simulink model "k1visitmyt"  (Simulink 8.6)
settings: Solver=ode45  StartTime=0.0  StopTime=10.0  RelTol=1e-3
libraries: cdsIPCx x21, cdsTP x5, cdsCDI64 x4, cdsCDO64 x4, BIO_CD_ENCODE_MASTER x4, BIO_CD_DECODE_MASTER x4, CHK_DIO x4, VIS_LIB x3, dac x2, cdsAdcx0 x1, cdsAdcx1 x1, cdsAdcx2 x1
settings Model: Creator=controls  LastModifiedBy=controls
settings DataIOCC: SignalLoggingSaveFormat=Dataset
settings OptimizationCC: ExpressionDepthLimit=128
settings DebuggingCC: UnderspecifiedInitializationDetection=Simplified  MergeDetectMultiDrivingBlocksExec=error  SolverPrmCheckMsg=none  FcnCallInpInsideContextMsg=EnableAllAsError  StateNameClashWarn=none
settings GRTTargetCC: CombineOutputUpdateFcns=on  GRTInterface=off

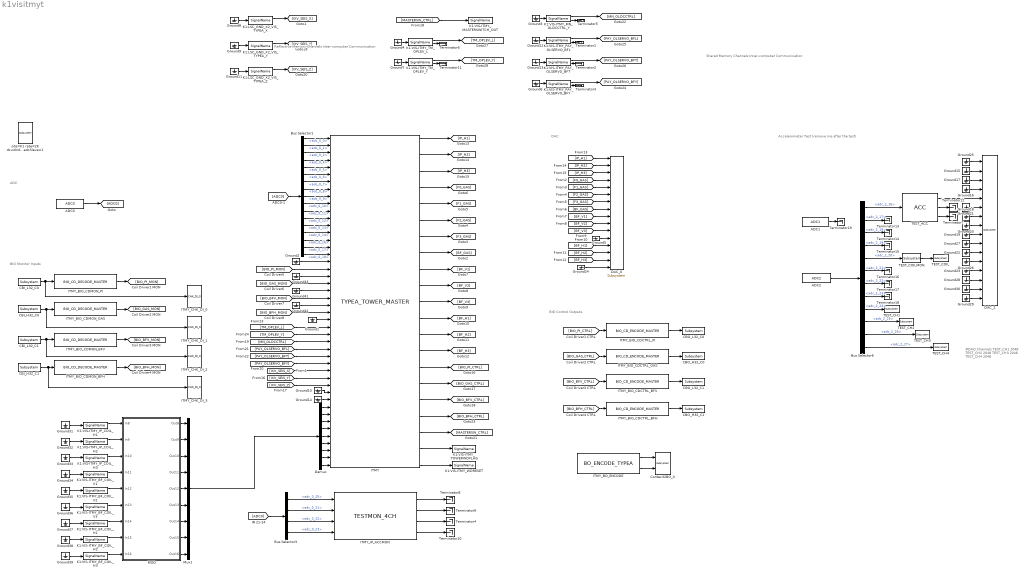
== system k1visitmyt ==
  note: BIO Monitor Inputs
  note: BIO Control Outputs
  note: DAC
  note: ADC
  note: Reflective Memory Channels
      | Inter-computer Communication
  note: Shared Memory Channels
      | Inner-computer Communication
  note: Accelerometer Test (remove me after the test)
  note: #DAQ Channels
      |
      | TEST_CH1 2048
      | TEST_CH2 2048
      | TEST_CH3 2048
      | TEST_CH4 2048
  ADC0 : cdsAdcx0/ADC0  Tag=cdsAdc  Description=|
      | type-GSC_16AI64SSA
      | card_num=0
      settings: AttributesFormatString=%<Description>\n%<Tag>
  ADC1 : cdsAdcx1/ADC1  Tag=cdsAdc  Description=|
      | type-GSC_16AI64SSA
      | card_num=1
      settings: AttributesFormatString=%<Description>\n%<Tag>
  ADC2 : cdsAdcx2/ADC2  Tag=cdsAdc  Description=|
      | type-GSC_16AI64SSA
      | card_num=2
      settings: AttributesFormatString=%<Description>\n%<Tag>
  Bus Selector1 : BusSelector  OutputSignals=adc_0_0,adc_0_1,adc_0_2,adc_0_4,adc_0_5,adc_0_6,adc_0_7,adc_0_8,adc_0_9,adc_0_10,adc_0_11,adc_0_12,adc_0_13,adc_0_14,adc_0_16,adc_0_17,adc_0_18
  Bus Selector3 : BusSelector  OutputSignals=adc_0_20,adc_0_21,adc_0_22,adc_0_23
  Bus Selector6 : BusSelector  Description=ADC Selector  OutputSignals=adc_2_16,adc_2_17,adc_2_18,adc_2_19,adc_2_20,adc_2_21,adc_2_22,adc_2_23,adc_2_24,adc_2_25,adc_2_26,adc_2_27
      settings: AttributesFormatString=%<Description>
  CBI_H32_C0 : cdsCDI64/Subsystem  Tag=cdsCDI64  Description=card_num=1
      settings: AttributesFormatString=%<Tag>\n%<Description>
  CBI_H32_C1 : cdsCDI64/Subsystem  Tag=cdsCDI64  Description=card_num=3
      settings: AttributesFormatString=%<Tag>\n%<Description>
  CBI_L32_C0 : cdsCDI64/Subsystem  Tag=cdsCDI64  Description=card_num=0
      settings: AttributesFormatString=%<Tag>\n%<Description>
  CBI_L32_C1 : cdsCDI64/Subsystem  Tag=cdsCDI64  Description=card_num=2
      settings: AttributesFormatString=%<Tag>\n%<Description>
  CBO_H32_C0 : cdsCDO64/Subsystem  Tag=cdsCDO64  Description=card_num=1
      settings: AttributesFormatString=%<Tag>\n%<Description>
  CBO_H32_C1 : cdsCDO64/Subsystem  Tag=cdsCDO64  Description=card_num=3
      settings: AttributesFormatString=%<Tag>\n%<Description>
  CBO_L32_C0 : cdsCDO64/Subsystem  Tag=cdsCDO64  Description=card_num=0
      settings: AttributesFormatString=%<Tag>\n%<Description>
  CBO_L32_C1 : cdsCDO64/Subsystem  Tag=cdsCDO64  Description=card_num=2
      settings: AttributesFormatString=%<Tag>\n%<Description>
  Contec32BO_0 : cdsCDO32/Subsystem  Tag=cdsCDO32  Description=Contec32 bit binary output module driver
      settings: AttributesFormatString=%<Tag>
  DAC_0 : dac/Subsystem  Description=|
      | type=GSC_16AO16,
      | card_num=0
      settings: AttributesFormatString=%<Description>
  DAC_2 : dac/Subsystem  Description=|
      | type=GSC_16AO16,
      | card_num=2
      settings: AttributesFormatString=%<Description>
  Demux : Demux  Outputs=9
  Ground{1..39,41..43} (42 alike) : Ground
  ITMY : TYPEA_MASTER/TYPEA_TOWER_MASTER
  ITMY_BIO_CDCTRL_BFH : BIO_CD_ENCODE_MASTER/BIO_CD_ENCODE_MASTER
  ITMY_BIO_CDCTRL_BFV : BIO_CD_ENCODE_MASTER/BIO_CD_ENCODE_MASTER
  ITMY_BIO_CDCTRL_GAS : BIO_CD_ENCODE_MASTER/BIO_CD_ENCODE_MASTER
  ITMY_BIO_CDCTRL_PI : BIO_CD_ENCODE_MASTER/BIO_CD_ENCODE_MASTER
  ITMY_BIO_CDMON_BFH : BIO_CD_DECODE_MASTER/BIO_CD_DECODE_MASTER
  ITMY_BIO_CDMON_BFV : BIO_CD_DECODE_MASTER/BIO_CD_DECODE_MASTER
  ITMY_BIO_CDMON_GAS : BIO_CD_DECODE_MASTER/BIO_CD_DECODE_MASTER
  ITMY_BIO_CDMON_PI : BIO_CD_DECODE_MASTER/BIO_CD_DECODE_MASTER
  ITMY_BO_ENCODE : BO_TYPEA_MASTER/BO_ENCODE_TYPEA
  ITMY_CHK_DI_{0..3} (4 alike) : CHK_DIO/CHK_DI_0
  ITMY_IP_ACCMON : TESTMON_4CH_MASTER/TESTMON_4CH
  K1:LSC_GND_X2_VIS_TYPEA_X : cdsIPCx/SignalName  Tag=cdsIPCx_RFM  Description=card=1
      settings: AttributesFormatString=%<Description>\n%<Tag>
  K1:LSC_GND_X2_VIS_TYPEA_Y : cdsIPCx/SignalName  Tag=cdsIPCx_RFM  Description=card=1
      settings: AttributesFormatString=%<Description>\n%<Tag>
  K1:LSC_GND_X2_VIS_TYPEA_Z : cdsIPCx/SignalName  Tag=cdsIPCx_RFM  Description=card=1
      settings: AttributesFormatString=%<Description>\n%<Tag>
  K1:VIS-ITMY_BF_COIL_H1 : cdsIPCx/SignalName  Tag=cdsIPCx_SHMEM  Description=Inter-Process Communication via Shared memory.
      settings: AttributesFormatString=%<Tag>
  K1:VIS-ITMY_BF_COIL_H2 : cdsIPCx/SignalName  Tag=cdsIPCx_SHMEM  Description=Inter-Process Communication via Shared memory.
      settings: AttributesFormatString=%<Tag>
  K1:VIS-ITMY_BF_COIL_H3 : cdsIPCx/SignalName  Tag=cdsIPCx_SHMEM  Description=Inter-Process Communication via Shared memory.
      settings: AttributesFormatString=%<Tag>
  K1:VIS-ITMY_BF_COIL_V1 : cdsIPCx/SignalName  Tag=cdsIPCx_SHMEM  Description=Inter-Process Communication via Shared memory.
      settings: AttributesFormatString=%<Tag>
  K1:VIS-ITMY_BF_COIL_V2 : cdsIPCx/SignalName  Tag=cdsIPCx_SHMEM  Description=Inter-Process Communication via Shared memory.
      settings: AttributesFormatString=%<Tag>
  K1:VIS-ITMY_BF_COIL_V3 : cdsIPCx/SignalName  Tag=cdsIPCx_SHMEM  Description=Inter-Process Communication via Shared memory.
      settings: AttributesFormatString=%<Tag>
  K1:VIS-ITMY_IP_COIL_H1 : cdsIPCx/SignalName  Tag=cdsIPCx_SHMEM  Description=Inter-Process Communication via Shared memory.
      settings: AttributesFormatString=%<Tag>
  K1:VIS-ITMY_IP_COIL_H2 : cdsIPCx/SignalName  Tag=cdsIPCx_SHMEM  Description=Inter-Process Communication via Shared memory.
      settings: AttributesFormatString=%<Tag>
  K1:VIS-ITMY_IP_COIL_H3 : cdsIPCx/SignalName  Tag=cdsIPCx_SHMEM  Description=Inter-Process Communication via Shared memory.
      settings: AttributesFormatString=%<Tag>
  K1:VIS-ITMY_MASTERSWITCH_OUT : cdsIPCx/SignalName  Tag=cdsIPCx_SHMEM  Description=Inter-Process Communication via Shared memory.
      settings: AttributesFormatString=%<Tag>
  K1:VIS-ITMY_MN_OLDCCTRL_Y : cdsIPCx/SignalName  Tag=cdsIPCx_SHMEM  Description=Inter-Process Communication via Shared memory.
      settings: AttributesFormatString=%<Tag>
  K1:VIS-ITMY_PAY_OLSERVO_BFL : cdsIPCx/SignalName  Tag=cdsIPCx_SHMEM  Description=Inter-Process Communication via Shared memory.
      settings: AttributesFormatString=%<Tag>
  K1:VIS-ITMY_PAY_OLSERVO_BFT : cdsIPCx/SignalName  Tag=cdsIPCx_SHMEM  Description=Inter-Process Communication via Shared memory.
      settings: AttributesFormatString=%<Tag>
  K1:VIS-ITMY_PAY_OLSERVO_BFY : cdsIPCx/SignalName  Tag=cdsIPCx_SHMEM  Description=Inter-Process Communication via Shared memory.
      settings: AttributesFormatString=%<Tag>
  K1:VIS-ITMY_TM_OPLEV_L : cdsIPCx/SignalName  Tag=cdsIPCx_SHMEM  Description=Inter-Process Communication via Shared memory.
      settings: AttributesFormatString=%<Tag>
  K1:VIS-ITMY_TM_OPLEV_Y : cdsIPCx/SignalName  Tag=cdsIPCx_SHMEM  Description=Inter-Process Communication via Shared memory.
      settings: AttributesFormatString=%<Tag>
  K1:VIS-ITMY_TOWERWDFLAG : cdsIPCx/SignalName  Tag=cdsIPCx_SHMEM  Description=Inter-Process Communication via Shared memory.
      settings: AttributesFormatString=%<Tag>
  K1:VIS-ITMY_WDRESET : cdsIPCx/SignalName  Tag=cdsIPCx_SHMEM  Description=Inter-Process Communication via Shared memory.
      settings: AttributesFormatString=%<Tag>
  MOD : Subsystem  Tag=top_names
  Mux1 : Mux  Inputs=9
  TEST_ACC : VIS_LIB/ACC
  TEST_CH{1..4} (4 alike) : cdsTP/Subsystem  Tag=Test Point
      settings: AttributesFormatString=%<Tag>
  TEST_COIL : cdsTP/Subsystem  Tag=Test Point
      settings: AttributesFormatString=%<Tag>
  TEST_COILMON : cdsEpicsOut/Subsystem  Tag=cdsEpicsOutput  Description=|
      | Purpose:                                          
      | Output a FE signal to an EPICS channel.           
      |                                                   
      | Operation:                                        
      | Takes input value and passes it to EPICS record.  
      |                                                   
      | Usage:                                            
      | Name the part with the desired EPICS rrecord name.
      settings: AttributesFormatString=%<Tag>
  Terminator{1..19} (19 alike) : Terminator
  site=K1 rate=2K dcuid=62 host=k1iy1 specific_cpu=3 adcSlave=1 : cdsParameters/Subsystem  Tag=cdsParameters  Description=|
      | Purpose:                                                                                                                                                                                                                                
      | Provide system parameters to the FE code generator to properly configure the generated EPICS names, rep rate of the FE controller, and the Data Acquisition node ID for proper storage of data from this FE controller.                 
      |                                                                                                                                                                                                                                         
      | Useage:                                                                                                                                                                                                                                 
      | The part NAME field is used to identify the FE parameters. It must be of the form:                                                                                                                                                      
      | site=                                                                                                                                                                                                                                   
      | rate=                                                                                                                                                                                                                                   
      | dcuid=                                                                                                                                                                                                                                  
      |                                                                                                                                                                                                                                         
      | Where:                                                                                                                                                                                                                                  
      | site= argument may be H1, H2, L1, M1, G1, either as a single argument or multiple, for example site=H1,H2. These are the only names allowed. These will become the first two characters of all EPICS and signal names (for example G1:).
      |                                                                                                                                                                                                                                         
      | rate= may be 2K, 16K, 32K, or 64K                                                                                                                                                                                                       
      |                                                                                                                                                                                                                                         
      | dcuid= is site specific ie it must be unique at each site.
      settings: AttributesFormatString=%<Tag>
  wires:
  ADC0/1 -> [ADC0]
  ITMY/4 -> [F0_GAS]
  ITMY/5 -> [F1_GAS]
  ITMY/8 -> [BF_GAS]
  ITMY/7 -> [F3_GAS]
  ITMY/6 -> [F2_GAS]
  ITMY/9 -> [BF_V1]
  ITMY/10 -> [BF_V2]
  ITMY/11 -> [BF_V3]
  ITMY/12 -> [BF_H1]
  ITMY/13 -> [BF_H2]
  ITMY/14 -> [BF_H3]
  [BF_H2] -> DAC_0/14
  [BF_V3] -> DAC_0/11
  [BF_H3] -> DAC_0/15
  [BF_V1] -> DAC_0/9
  [BF_H1] -> DAC_0/13
  [BF_V2] -> DAC_0/10
  ITMY/1 -> [IP_H1]
  ITMY/2 -> [IP_H2]
  ITMY/3 -> [IP_H3]
  CBI_H32_C0/1 -> ITMY_CHK_DI_1/1, ITMY_BIO_CDMON_GAS/1
  CBI_L32_C1/1 -> ITMY_CHK_DI_2/1, ITMY_BIO_CDMON_BFV/1
  CBI_L32_C0/1 -> ITMY_CHK_DI_0/1, ITMY_BIO_CDMON_PI/1
  CBI_H32_C1/1 -> ITMY_CHK_DI_3/1, ITMY_BIO_CDMON_BFH/1
  ITMY_BIO_CDCTRL_BFH/1 -> CBO_H32_C1/1
  ITMY_BIO_CDCTRL_PI/1 -> CBO_L32_C0/1
  ITMY_BIO_CDCTRL_GAS/1 -> CBO_H32_C0/1
  ITMY_BIO_CDCTRL_BFV/1 -> CBO_L32_C1/1
  [BIO_PI_CTRL] -> ITMY_BIO_CDCTRL_PI/1
  [BIO_GAS_CTRL] -> ITMY_BIO_CDCTRL_GAS/1
  [BIO_BFV_CTRL] -> ITMY_BIO_CDCTRL_BFV/1
  ITMY_BIO_CDMON_PI/1 -> [BIO_PI_MON]
  ITMY_BIO_CDMON_GAS/1 -> [BIO_GAS_MON]
  ITMY_BIO_CDMON_BFH/1 -> [BIO_BFH_MON]
  ITMY_BIO_CDMON_BFV/1 -> [BIO_BFV_MON]
  [BIO_BFH_CTRL] -> ITMY_BIO_CDCTRL_BFH/1
  [IP_H1] -> DAC_0/1
  [IP_H2] -> DAC_0/2
  [IP_H3] -> DAC_0/3
  [F0_GAS] -> DAC_0/4
  [F1_GAS] -> DAC_0/5
  [F2_GAS] -> DAC_0/6
  [F3_GAS] -> DAC_0/7
  [BF_GAS] -> DAC_0/8
  [ADC0] -> Bus Selector3/1
  Bus Selector3/2 -> ITMY_IP_ACCMON/2  "<adc_0_21>"
  Bus Selector3/1 -> ITMY_IP_ACCMON/1  "<adc_0_20>"
  Bus Selector3/3 -> ITMY_IP_ACCMON/3  "<adc_0_22>"
  Bus Selector3/4 -> ITMY_IP_ACCMON/4  "<adc_0_23>"
  ITMY_IP_ACCMON/3 -> Terminator4/1
  ITMY_IP_ACCMON/4 -> Terminator10/1
  ITMY_IP_ACCMON/1 -> Terminator8/1
  ITMY_IP_ACCMON/2 -> Terminator9/1
  Ground5/1 -> DAC_0/12
  Ground24/1 -> DAC_0/16
  ITMY/15 -> [BIO_PI_CTRL]
  ITMY/16 -> [BIO_GAS_CTRL]
  ITMY/17 -> [BIO_BFV_CTRL]
  ITMY/18 -> [BIO_BFH_CTRL]
  ITMY_BO_ENCODE/1 -> Contec32BO_0/1
  ITMY_BO_ENCODE/2 -> Contec32BO_0/2
  [ADC0] -> Bus Selector1/1
  Bus Selector1/1 -> ITMY/1  "<adc_0_0>"
  Bus Selector1/2 -> ITMY/2  "<adc_0_1>"
  Bus Selector1/3 -> ITMY/3  "<adc_0_2>"
  Bus Selector1/4 -> ITMY/4  "<adc_0_4>"
  Bus Selector1/5 -> ITMY/5  "<adc_0_5>"
  Bus Selector1/6 -> ITMY/6  "<adc_0_6>"
  Bus Selector1/7 -> ITMY/7  "<adc_0_7>"
  Bus Selector1/8 -> ITMY/8  "<adc_0_8>"
  Bus Selector1/9 -> ITMY/9  "<adc_0_9>"
  Bus Selector1/10 -> ITMY/10  "<adc_0_10>"
  Bus Selector1/11 -> ITMY/11  "<adc_0_11>"
  Bus Selector1/12 -> ITMY/12  "<adc_0_12>"
  Bus Selector1/13 -> ITMY/13  "<adc_0_13>"
  Bus Selector1/14 -> ITMY/14  "<adc_0_14>"
  Bus Selector1/15 -> ITMY/15  "<adc_0_16>"
  Bus Selector1/16 -> ITMY/16  "<adc_0_17>"
  Bus Selector1/17 -> ITMY/17  "<adc_0_18>"
  [BIO_PI_MON] -> ITMY/19
  [BIO_GAS_MON] -> ITMY/21
  [BIO_BFV_MON] -> ITMY/23
  [BIO_BFH_MON] -> ITMY/25
  Ground43/1 -> ITMY/20
  Ground41/1 -> ITMY/22
  Ground42/1 -> ITMY/24
  Ground2/1 -> ITMY/18
  Ground8/1 -> K1:LSC_GND_X2_VIS_TYPEA_X/1
  Ground9/1 -> K1:LSC_GND_X2_VIS_TYPEA_Y/1
  Ground11/1 -> K1:LSC_GND_X2_VIS_TYPEA_Z/1
  K1:LSC_GND_X2_VIS_TYPEA_X/1 -> [IXV_SEIS_X]
  K1:LSC_GND_X2_VIS_TYPEA_Y/1 -> [IXV_SEIS_Y]
  K1:LSC_GND_X2_VIS_TYPEA_Z/1 -> [IXV_SEIS_Z]
  K1:VIS-ITMY_PAY_OLSERVO_BFY/2 -> Terminator3/1
  K1:VIS-ITMY_MN_OLDCCTRL_Y/2 -> Terminator5/1
  Ground3/1 -> K1:VIS-ITMY_MN_OLDCCTRL_Y/1
  Ground6/1 -> K1:VIS-ITMY_PAY_OLSERVO_BFY/1
  K1:VIS-ITMY_PAY_OLSERVO_BFY/1 -> [PAY_OLSERVO_BFY]
  K1:VIS-ITMY_MN_OLDCCTRL_Y/1 -> [MN_OLDCCTRL]
  K1:VIS-ITMY_PAY_OLSERVO_BFL/2 -> Terminator1/1
  Ground12/1 -> K1:VIS-ITMY_PAY_OLSERVO_BFL/1
  K1:VIS-ITMY_PAY_OLSERVO_BFL/1 -> [PAY_OLSERVO_BFL]
  K1:VIS-ITMY_PAY_OLSERVO_BFT/2 -> Terminator2/1
  Ground13/1 -> K1:VIS-ITMY_PAY_OLSERVO_BFT/1
  K1:VIS-ITMY_PAY_OLSERVO_BFT/1 -> [PAY_OLSERVO_BFT]
  K1:VIS-ITMY_TM_OPLEV_L/2 -> Terminator6/1
  Ground4/1 -> K1:VIS-ITMY_TM_OPLEV_L/1
  K1:VIS-ITMY_TM_OPLEV_L/1 -> [TM_OPLEV_L]
  K1:VIS-ITMY_TM_OPLEV_Y/2 -> Terminator11/1
  Ground7/1 -> K1:VIS-ITMY_TM_OPLEV_Y/1
  K1:VIS-ITMY_TM_OPLEV_Y/1 -> [TM_OPLEV_Y]
  ITMY/21 -> K1:VIS-ITMY_WDRESET/1
  ITMY/20 -> K1:VIS-ITMY_TOWERWDFLAG/1
  ITMY/19 -> [MASTERSW_CTRL]
  [MASTERSW_CTRL] -> K1:VIS-ITMY_MASTERSWITCH_OUT/1
  Ground14/1 -> ITMY/37
  Ground10/1 -> ITMY/36
  [IXV_SEIS_Z] -> ITMY/35
  [IXV_SEIS_Y] -> ITMY/34
  [IXV_SEIS_X] -> ITMY/33
  [PAY_OLSERVO_BFY] -> ITMY/32
  [PAY_OLSERVO_BFT] -> ITMY/31
  [PAY_OLSERVO_BFL] -> ITMY/30
  [MN_OLDCCTRL] -> ITMY/29
  [TM_OPLEV_Y] -> ITMY/28
  [TM_OPLEV_L] -> ITMY/27
  Ground1/1 -> ITMY/26
  Ground25/1 -> DAC_2/1
  Ground15/1 -> DAC_2/2
  Ground16/1 -> DAC_2/4
  Ground17/1 -> DAC_2/3
  ADC2/1 -> Bus Selector6/1
  Bus Selector6/1 -> TEST_ACC/1  "<adc_2_16>"
  TEST_ACC/1 -> DAC_2/5
  TEST_ACC/3 -> Terminator7/1
  TEST_ACC/2 -> Terminator12/1
  Ground18/1 -> DAC_2/7
  Ground21/1 -> DAC_2/6
  Ground20/1 -> DAC_2/8
  Ground19/1 -> DAC_2/9
  Ground27/1 -> DAC_2/10
  Ground22/1 -> DAC_2/11
  Ground26/1 -> DAC_2/12
  Ground23/1 -> DAC_2/13
  Ground28/1 -> DAC_2/14
  Ground30/1 -> DAC_2/15
  Ground29/1 -> DAC_2/16
  TEST_COILMON/1 -> TEST_COIL/1
  Bus Selector6/5 -> TEST_COILMON/1  "<adc_2_20>"
  Bus Selector6/2 -> Terminator13/1  "<adc_2_17>"
  Bus Selector6/3 -> Terminator14/1  "<adc_2_18>"
  Bus Selector6/4 -> Terminator15/1  "<adc_2_19>"
  Bus Selector6/9 -> TEST_CH1/1  "<adc_2_24>"
  Bus Selector6/10 -> TEST_CH2/1  "<adc_2_25>"
  Bus Selector6/6 -> Terminator16/1  "<adc_2_21>"
  Bus Selector6/7 -> Terminator17/1  "<adc_2_22>"
  Bus Selector6/8 -> Terminator18/1  "<adc_2_23>"
  Bus Selector6/11 -> TEST_CH3/1  "<adc_2_26>"
  Bus Selector6/12 -> TEST_CH4/1  "<adc_2_27>"
  ADC1/1 -> Terminator19/1
  Ground31/1 -> K1:VIS-ITMY_IP_COIL_H1/1
  K1:VIS-ITMY_IP_COIL_H1/1 -> MOD/1(In8)
  K1:VIS-ITMY_BF_COIL_H3/1 -> MOD/9(In16)
  K1:VIS-ITMY_IP_COIL_H2/1 -> MOD/2(In9)
  K1:VIS-ITMY_IP_COIL_H3/1 -> MOD/3(In10)
  K1:VIS-ITMY_BF_COIL_V1/1 -> MOD/4(In11)
  K1:VIS-ITMY_BF_COIL_V2/1 -> MOD/5(In12)
  K1:VIS-ITMY_BF_COIL_V3/1 -> MOD/6(In13)
  K1:VIS-ITMY_BF_COIL_H1/1 -> MOD/7(In14)
  K1:VIS-ITMY_BF_COIL_H2/1 -> MOD/8(In15)
  Ground32/1 -> K1:VIS-ITMY_IP_COIL_H2/1
  Ground33/1 -> K1:VIS-ITMY_IP_COIL_H3/1
  Ground34/1 -> K1:VIS-ITMY_BF_COIL_V1/1
  Ground35/1 -> K1:VIS-ITMY_BF_COIL_V2/1
  Ground36/1 -> K1:VIS-ITMY_BF_COIL_V3/1
  Ground37/1 -> K1:VIS-ITMY_BF_COIL_H1/1
  Ground38/1 -> K1:VIS-ITMY_BF_COIL_H2/1
  Ground39/1 -> K1:VIS-ITMY_BF_COIL_H3/1
  MOD/1(Out8) -> Mux1/1
  MOD/2(Out9) -> Mux1/2
  MOD/3(Out10) -> Mux1/3
  MOD/4(Out11) -> Mux1/4
  MOD/5(Out12) -> Mux1/5
  MOD/6(Out13) -> Mux1/6
  MOD/7(Out14) -> Mux1/7
  MOD/8(Out15) -> Mux1/8
  MOD/9(Out16) -> Mux1/9
  Demux/1 -> ITMY/38
  Demux/2 -> ITMY/39
  Demux/3 -> ITMY/40
  Demux/4 -> ITMY/41
  Demux/5 -> ITMY/42
  Demux/6 -> ITMY/43
  Demux/7 -> ITMY/44
  Demux/8 -> ITMY/45
  Demux/9 -> ITMY/46
  Mux1/1 -> Demux/1

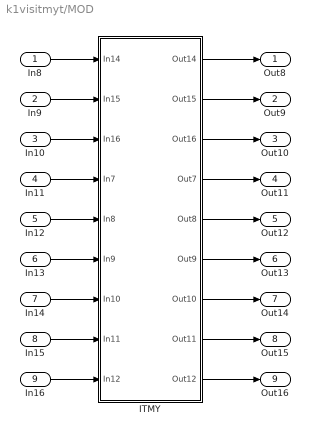
== system k1visitmyt/MOD ==
  In8 : Inport
  In9 : Inport  Port=2
  In10 : Inport  Port=3
  In11 : Inport  Port=4
  In12 : Inport  Port=5
  In13 : Inport  Port=6
  In14 : Inport  Port=7
  In15 : Inport  Port=8
  In16 : Inport  Port=9
  ITMY : Subsystem
  Out8 : Outport
  Out9 : Outport  Port=2
  Out10 : Outport  Port=3
  Out11 : Outport  Port=4
  Out12 : Outport  Port=5
  Out13 : Outport  Port=6
  Out14 : Outport  Port=7
  Out15 : Outport  Port=8
  Out16 : Outport  Port=9
  wires:
  ITMY/9(Out12) -> Out16/1
  ITMY/1(Out14) -> Out8/1
  ITMY/2(Out15) -> Out9/1
  ITMY/3(Out16) -> Out10/1
  ITMY/4(Out7) -> Out11/1
  ITMY/5(Out8) -> Out12/1
  ITMY/6(Out9) -> Out13/1
  ITMY/7(Out10) -> Out14/1
  ITMY/8(Out11) -> Out15/1
  In8/1 -> ITMY/1(In14)
  In9/1 -> ITMY/2(In15)
  In10/1 -> ITMY/3(In16)
  In11/1 -> ITMY/4(In7)
  In12/1 -> ITMY/5(In8)
  In13/1 -> ITMY/6(In9)
  In14/1 -> ITMY/7(In10)
  In15/1 -> ITMY/8(In11)
  In16/1 -> ITMY/9(In12)

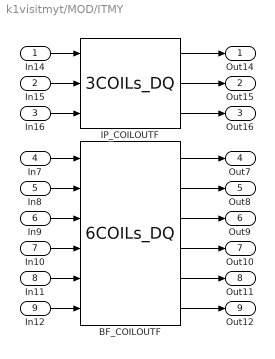
== system k1visitmyt/MOD/ITMY ==
  In14 : Inport
  In15 : Inport  Port=2
  In16 : Inport  Port=3
  In7 : Inport  Port=4
  In8 : Inport  Port=5
  In9 : Inport  Port=6
  In10 : Inport  Port=7
  In11 : Inport  Port=8
  In12 : Inport  Port=9
  BF_COILOUTF : VIS_LIB/UTILs/6COILs_DQ
  IP_COILOUTF : VIS_LIB/UTILs/3COILs_DQ
  Out14 : Outport
  Out15 : Outport  Port=2
  Out16 : Outport  Port=3
  Out7 : Outport  Port=4
  Out8 : Outport  Port=5
  Out9 : Outport  Port=6
  Out10 : Outport  Port=7
  Out11 : Outport  Port=8
  Out12 : Outport  Port=9
  wires:
  In16/1 -> IP_COILOUTF/3
  IP_COILOUTF/2 -> Out15/1
  In14/1 -> IP_COILOUTF/1
  In15/1 -> IP_COILOUTF/2
  IP_COILOUTF/1 -> Out14/1
  IP_COILOUTF/3 -> Out16/1
  In10/1 -> BF_COILOUTF/4
  BF_COILOUTF/1 -> Out7/1
  BF_COILOUTF/3 -> Out9/1
  In11/1 -> BF_COILOUTF/5
  In7/1 -> BF_COILOUTF/1
  In8/1 -> BF_COILOUTF/2
  In9/1 -> BF_COILOUTF/3
  BF_COILOUTF/5 -> Out11/1
  BF_COILOUTF/6 -> Out12/1
  In12/1 -> BF_COILOUTF/6
  BF_COILOUTF/2 -> Out8/1
  BF_COILOUTF/4 -> Out10/1
